simulink model "Simulink_simulation"  (R2019b)
settings: Solver=VariableStepAuto  StartTime=0.0  StopTime=10.0  RelTol=1e-3
undefined symbols (not defined in the file or in its folder): bottom1, bottom2, C1_feed, Dist_1, Dist_2, overall_Feed, X_Eth_feed1, X_FEED_Eth, X_FEED_Wat, X_Wat_feed1, XB1_Eth, XB1_water, XB2_Eth, XB2_Wat, Xd1, XD1_Wat, Xd2, XD2_Wat
settings Model: Creator=PE-Ma  LastModifiedBy=PE-Ma

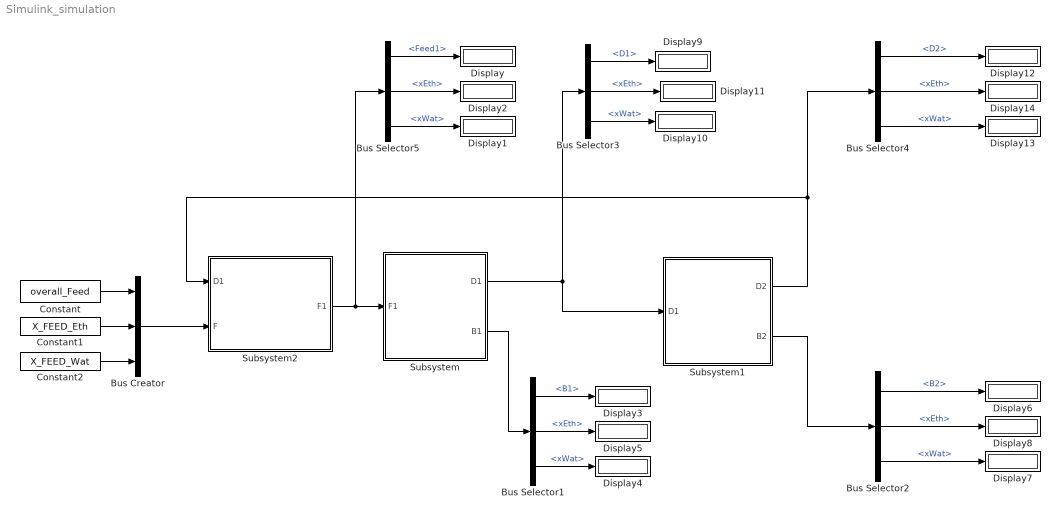
== system Simulink_simulation ==
  Bus Creator : BusCreator  Inputs=3
  Bus Selector1 : BusSelector  OutputSignals=B1,xEth,xWat
  Bus Selector2 : BusSelector  OutputSignals=B2,xEth,xWat
  Bus Selector3 : BusSelector  OutputSignals=D1,xEth,xWat
  Bus Selector4 : BusSelector  OutputSignals=D2,xEth,xWat
  Bus Selector5 : BusSelector  OutputSignals=Feed1,xEth,xWat
  Constant : Constant  Value=overall_Feed
  Constant1 : Constant  Value=X_FEED_Eth
  Constant2 : Constant  Value=X_FEED_Wat
  Display{,1..14} (15 alike) : Display
  Subsystem : Subsystem
      mask Display: image('$imagefile'); % Use "Edit Image" on toolstrip to change.
  Subsystem1 : Subsystem
      mask Display: image('$imagefile'); % Use "Edit Image" on toolstrip to change.
  Subsystem2 : Subsystem
      mask Display: image('$imagefile'); % Use "Edit Image" on toolstrip to change.
  wires:
  Constant1/1 -> Bus Creator/2
  Constant/1 -> Bus Creator/1
  Constant2/1 -> Bus Creator/3
  Bus Creator/1 -> Subsystem2/2(F)
  Subsystem2/1(F1) -> Bus Selector5/1, Subsystem/1(F1)
  Bus Selector5/1 -> Display/1  "<Feed1>"
  Bus Selector5/2 -> Display2/1  "<xEth>"
  Bus Selector5/3 -> Display1/1  "<xWat>"
  Bus Selector1/3 -> Display4/1  "<xWat>"
  Subsystem/2(B1) -> Bus Selector1/1
  Bus Selector1/1 -> Display3/1  "<B1>"
  Bus Selector1/2 -> Display5/1  "<xEth>"
  Bus Selector2/2 -> Display8/1  "<xEth>"
  Subsystem1/2(B2) -> Bus Selector2/1
  Bus Selector2/1 -> Display6/1  "<B2>"
  Bus Selector2/3 -> Display7/1  "<xWat>"
  Bus Selector3/3 -> Display10/1  "<xWat>"
  Bus Selector3/1 -> Display9/1  "<D1>"
  Bus Selector3/2 -> Display11/1  "<xEth>"
  Subsystem/1(D1) -> Subsystem1/1(D1), Bus Selector3/1
  Bus Selector4/3 -> Display13/1  "<xWat>"
  Bus Selector4/1 -> Display12/1  "<D2>"
  Bus Selector4/2 -> Display14/1  "<xEth>"
  Subsystem1/1(D2) -> Subsystem2/1(D1), Bus Selector4/1

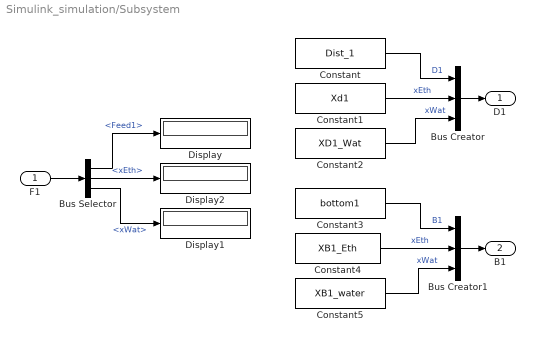
== system Simulink_simulation/Subsystem ==
  F1 : Inport
  Bus Creator : BusCreator  Inputs=3
  Bus Creator1 : BusCreator  Inputs=3
  Bus Selector : BusSelector  OutputSignals=Feed1,xEth,xWat
  Constant : Constant  Value=Dist_1
  Constant1 : Constant  Value=Xd1
  Constant2 : Constant  Value=XD1_Wat
  Constant3 : Constant  Value=bottom1
  Constant4 : Constant  Value=XB1_Eth
  Constant5 : Constant  Value=XB1_water
  Display : Display
  Display1 : Display
  Display2 : Display
  D1 : Outport
  B1 : Outport  Port=2
  wires:
  F1/1 -> Bus Selector/1
  Bus Selector/1 -> Display/1  "<Feed1>"
  Bus Selector/3 -> Display1/1  "<xWat>"
  Bus Selector/2 -> Display2/1  "<xEth>"
  Constant2/1 -> Bus Creator/3  "xWat"
  Constant1/1 -> Bus Creator/2  "xEth"
  Constant/1 -> Bus Creator/1  "D1"
  Constant4/1 -> Bus Creator1/2  "xEth"
  Constant3/1 -> Bus Creator1/1  "B1"
  Constant5/1 -> Bus Creator1/3  "xWat"
  Bus Creator/1 -> D1/1
  Bus Creator1/1 -> B1/1

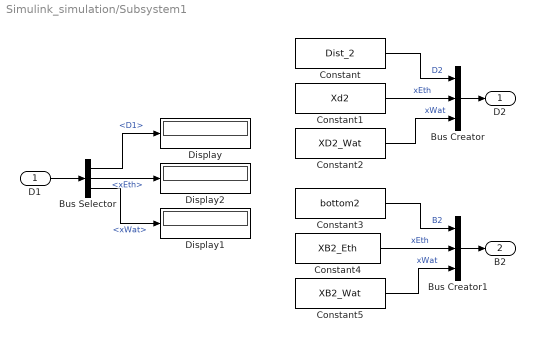
== system Simulink_simulation/Subsystem1 ==
  D1 : Inport
  Bus Creator : BusCreator  Inputs=3
  Bus Creator1 : BusCreator  Inputs=3
  Bus Selector : BusSelector  OutputSignals=D1,xEth,xWat
  Constant : Constant  Value=Dist_2
  Constant1 : Constant  Value=Xd2
  Constant2 : Constant  Value=XD2_Wat
  Constant3 : Constant  Value=bottom2
  Constant4 : Constant  Value=XB2_Eth
  Constant5 : Constant  Value=XB2_Wat
  Display : Display
  Display1 : Display
  Display2 : Display
  D2 : Outport
  B2 : Outport  Port=2
  wires:
  D1/1 -> Bus Selector/1
  Bus Selector/1 -> Display/1  "<D1>"
  Bus Selector/3 -> Display1/1  "<xWat>"
  Bus Selector/2 -> Display2/1  "<xEth>"
  Constant2/1 -> Bus Creator/3  "xWat"
  Constant1/1 -> Bus Creator/2  "xEth"
  Constant/1 -> Bus Creator/1  "D2"
  Constant4/1 -> Bus Creator1/2  "xEth"
  Constant3/1 -> Bus Creator1/1  "B2"
  Constant5/1 -> Bus Creator1/3  "xWat"
  Bus Creator/1 -> D2/1
  Bus Creator1/1 -> B2/1

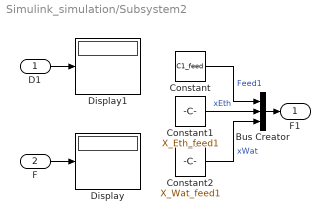
== system Simulink_simulation/Subsystem2 ==
  D1 : Inport
  F : Inport  Port=2
  Bus Creator : BusCreator  Inputs=3
  Constant : Constant  Value=C1_feed
  Constant1 : Constant  Value=X_Eth_feed1
  Constant2 : Constant  Value=X_Wat_feed1
  Display : Display
  Display1 : Display
  F1 : Outport
  wires:
  F/1 -> Display/1
  D1/1 -> Display1/1
  Constant1/1 -> Bus Creator/2  "xEth"
  Bus Creator/1 -> F1/1
  Constant/1 -> Bus Creator/1  "Feed1"
  Constant2/1 -> Bus Creator/3  "xWat"
